simulink model "double_pendulum_model_2D"  (R2021a)
settings: Solver=FixedStepAuto  StartTime=0.0  StopTime=10.0  RelTol=1e-3
undefined symbols (not defined in the file): c1, c2, Cdp, g, l1, l2, mp1, mp2, mq, rho
settings Model: Creator=francois  LastModifiedBy=esl
settings SolverCC: AlgebraicLoopSolver=TrustRegion
settings DebuggingCC: SFMachineParentedDataDiag=warning

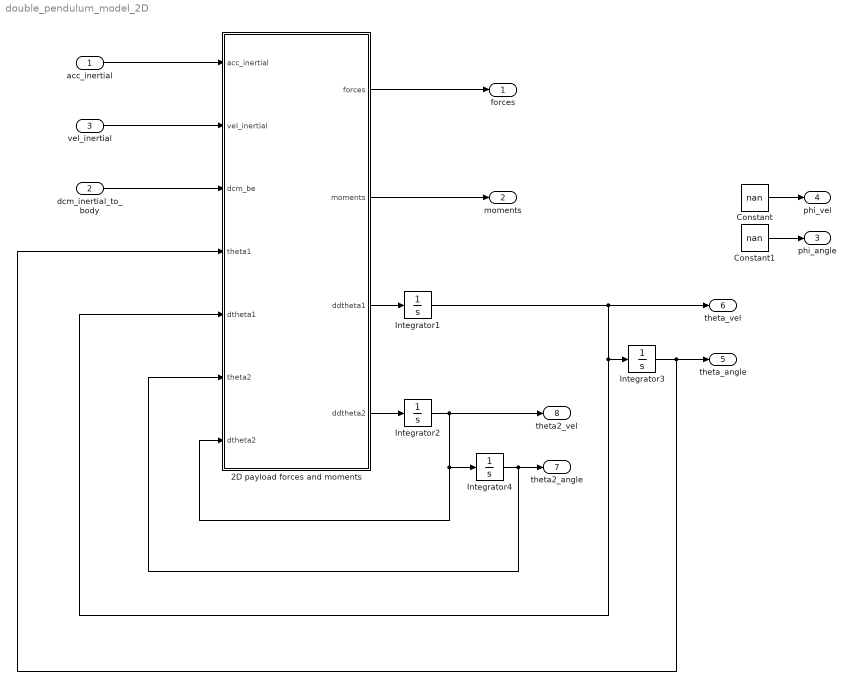
== system double_pendulum_model_2D ==
  acc_inertial : Inport  PortDimensions=3
  dcm_inertial_to_body : Inport  Port=2  PortDimensions=[3, 3]
  vel_inertial : Inport  Port=3  PortDimensions=3
  2D payload forces and moments : MATLAB Function  TreatAsAtomicUnit=on
  Constant : Constant  Value=nan
  Constant1 : Constant  Value=nan
  Integrator1 : Integrator
  Integrator2 : Integrator
  Integrator3 : Integrator  WrapState=on
  Integrator4 : Integrator  WrapState=on
  forces : Outport  PortDimensions=3
  moments : Outport  Port=2  PortDimensions=3
  phi_angle : Outport  Port=3  PortDimensions=1
  phi_vel : Outport  Port=4  PortDimensions=1
  theta_angle : Outport  Port=5  PortDimensions=1
  theta_vel : Outport  Port=6  PortDimensions=1
  theta2_angle : Outport  Port=7  PortDimensions=1
  theta2_vel : Outport  Port=8  PortDimensions=1
  wires:
  acc_inertial/1 -> 2D payload forces and moments/1(acc_inertial)
  dcm_inertial_to_body/1 -> 2D payload forces and moments/3(dcm_be)
  2D payload forces and moments/1(forces) -> forces/1
  Integrator1/1 -> 2D payload forces and moments/5(dtheta1), Integrator3/1, theta_vel/1
  2D payload forces and moments/3(ddtheta1) -> Integrator1/1
  Integrator3/1 -> 2D payload forces and moments/4(theta1), theta_angle/1
  2D payload forces and moments/2(moments) -> moments/1
  vel_inertial/1 -> 2D payload forces and moments/2(vel_inertial)
  Constant/1 -> phi_vel/1
  Constant1/1 -> phi_angle/1
  2D payload forces and moments/4(ddtheta2) -> Integrator2/1
  Integrator2/1 -> theta2_vel/1, 2D payload forces and moments/7(dtheta2), Integrator4/1
  Integrator4/1 -> 2D payload forces and moments/6(theta2), theta2_angle/1

== matlab function double_pendulum_model_2D/2D payload forces and moments ==
  data: acc_inertial input; vel_inertial input; forces output; dcm_be input; theta1 input; dtheta1 input; theta2 input; dtheta2 input; moments output; ddtheta1 output; ddtheta2 output; mq parameter; mp1 parameter; mp2 parameter; l1 parameter; l2 parameter; g parameter; c1 parameter; c2 parameter; Cdp parameter; rho parameter
function [forces, moments, ddtheta1 , ddtheta2] = double_pendulum_2D(acc_inertial, vel_inertial, dcm_be, theta1, dtheta1, theta2, dtheta2, mq, mp1, mp2, l1, l2, g, c1, c2, Cdp, rho)
    % all forces and states are relative to inertial frame coordinate frame
    
    % For variables used from MATLAB workspace, add them as function inputs
    % go to tab: "Editor", in section "SIMULINK", click "Edit Data"
    % for appropriate input args that are in MATLAB workspace, change scope
    % from "Input" to "Parameter"
    
    %% Drag forces
    fwt1 = (0.5*rho*(0 - ( vel_inertial(1) + dtheta1*l1*cos(theta1)                          ))^2*Cdp)*sign(vel_inertial(1));
    fwt2 = (0.5*rho*(0 - ( vel_inertial(1) + dtheta1*l1*cos(theta1) + dtheta2*l2*cos(theta2) ))^2*Cdp)*sign(vel_inertial(1));
    
    %% Quad acceleration    due to    actual payload angle and angular rate   
    % copy output from "calculate_double_pendulum_forces.m":
    ax = (2*fwt1*l1*l2*mp1^2 + 4*c1*dtheta1*l2*mp1^2*cos(theta1) + 2*fwt1*l1*l2*mp1*mp2 + 2*fwt1*l1*l2*mp1*mq + fwt1*l1*l2*mp2*mq + fwt2*l1*l2*mp1*mq + fwt2*l1*l2*mp2*mq + 2*fwt1*l1*l2*mp1^2*cos(2*theta1) + 2*g*l1*l2*mp1^2*mq*sin(2*theta1) + 4*c1*dtheta1*l2*mp1*mp2*cos(theta1) + 4*c1*dtheta1*l2*mp1*mq*cos(theta1) + 2*c1*dtheta1*l2*mp2*mq*cos(theta1) - 2*c2*dtheta1*l1*mp1*mq*cos(theta2) - 2*c2*dtheta1*l1*mp2*mq*cos(theta2) + 2*c2*dtheta2*l1*mp1*mq*cos(theta2) + 2*c2*dtheta2*l1*mp2*mq*cos(theta2) - 2*c1*dtheta1*l2*mp2*mq*cos(theta1 - 2*theta2) + 4*dtheta1^2*l1^2*l2*mp1^2*mq*sin(theta1) + 2*fwt1*l1*l2*mp1*mp2*cos(2*theta1) + 2*fwt1*l1*l2*mp1*mq*cos(2*theta1) + fwt1*l1*l2*mp2*mq*cos(2*theta1) - fwt2*l1*l2*mp1*mq*cos(2*theta1) - fwt1*l1*l2*mp2*mq*cos(2*theta2) + fwt2*l1*l2*mp1*mq*cos(2*theta2) - fwt2*l1*l2*mp2*mq*cos(2*theta1) + fwt2*l1*l2*mp2*mq*cos(2*theta2) + 2*c2*dtheta1*l1*mp1*mq*cos(2*theta1 - theta2) + 2*c2*dtheta1*l1*mp2*mq*cos(2*theta1 - theta2) - 2*c2*dtheta2*l1*mp1*mq*cos(2*theta1 - theta2) - 2*c2*dtheta2*l1*mp2*mq*cos(2*theta1 - theta2) - fwt1*l1*l2*mp2*mq*cos(2*theta1 - 2*theta2) - fwt2*l1*l2*mp1*mq*cos(2*theta1 - 2*theta2) - fwt2*l1*l2*mp2*mq*cos(2*theta1 - 2*theta2) + 2*dtheta2^2*l1*l2^2*mp1*mp2*mq*sin(2*theta1 - theta2) + 2*g*l1*l2*mp1*mp2*mq*sin(2*theta1) + 4*dtheta1^2*l1^2*l2*mp1*mp2*mq*sin(theta1) + 2*dtheta2^2*l1*l2^2*mp1*mp2*mq*sin(theta2))/(2*l1*l2*mq*(2*mp1*mp2 + 2*mp1*mq + mp2*mq + 2*mp1^2 - mp2*mq*cos(2*theta1 - 2*theta2)));
    az = (2*g*l1*l2*mp1^2*mq - 2*fwt1*l1*l2*mp1^2*sin(2*theta1) - 4*c1*dtheta1*l2*mp1^2*sin(theta1) + 2*g*l1*l2*mp1^2*mq*cos(2*theta1) - 4*c1*dtheta1*l2*mp1*mp2*sin(theta1) - 4*c1*dtheta1*l2*mp1*mq*sin(theta1) - 2*c1*dtheta1*l2*mp2*mq*sin(theta1) + 2*c2*dtheta1*l1*mp1*mq*sin(theta2) + 2*c2*dtheta1*l1*mp2*mq*sin(theta2) - 2*c2*dtheta2*l1*mp1*mq*sin(theta2) - 2*c2*dtheta2*l1*mp2*mq*sin(theta2) + 4*dtheta1^2*l1^2*l2*mp1^2*mq*cos(theta1) - 2*c1*dtheta1*l2*mp2*mq*sin(theta1 - 2*theta2) - 2*fwt1*l1*l2*mp1*mp2*sin(2*theta1) - 2*fwt1*l1*l2*mp1*mq*sin(2*theta1) - fwt1*l1*l2*mp2*mq*sin(2*theta1) + fwt2*l1*l2*mp1*mq*sin(2*theta1) + fwt1*l1*l2*mp2*mq*sin(2*theta2) - fwt2*l1*l2*mp1*mq*sin(2*theta2) + fwt2*l1*l2*mp2*mq*sin(2*theta1) - fwt2*l1*l2*mp2*mq*sin(2*theta2) + 2*g*l1*l2*mp1*mp2*mq - 2*c2*dtheta1*l1*mp1*mq*sin(2*theta1 - theta2) - 2*c2*dtheta1*l1*mp2*mq*sin(2*theta1 - theta2) + 2*c2*dtheta2*l1*mp1*mq*sin(2*theta1 - theta2) + 2*c2*dtheta2*l1*mp2*mq*sin(2*theta1 - theta2) - fwt1*l1*l2*mp2*mq*sin(2*theta1 - 2*theta2) + fwt2*l1*l2*mp1*mq*sin(2*theta1 - 2*theta2) + fwt2*l1*l2*mp2*mq*sin(2*theta1 - 2*theta2) + 2*dtheta2^2*l1*l2^2*mp1*mp2*mq*cos(2*theta1 - theta2) + 2*g*l1*l2*mp1*mp2*mq*cos(2*theta1) + 4*dtheta1^2*l1^2*l2*mp1*mp2*mq*cos(theta1) + 2*dtheta2^2*l1*l2^2*mp1*mp2*mq*cos(theta2))/(2*l1*l2*mq*(2*mp1*mp2 + 2*mp1*mq + mp2*mq + 2*mp1^2 - mp2*mq*cos(2*theta1 - 2*theta2)));

    ay = 0; % No y effect because using a 2D model
    
    %% Forces and moments based on payload contribution to acceleration
    forces = (mq + mp1 + mp2) * dcm_be * [ax; ay; az];
    moments = [0; 0; 0]; % No effect on moments
    
    %% Extract actual quad acceleration
    ddxq = acc_inertial(1);
%     ddy = acc_inertial(2); % No y effect because using a 2D model
    ddzq = acc_inertial(3);
        
    %% Payload angular acceleration,     due to    actual quad acceleration 
    % copy output from "calculate_double_pendulum_forces.m":
    ddtheta1 = -(c1*dtheta1*l2 + fwt1*l1*l2*cos(theta1) + c2*dtheta1*l1*cos(theta1 - theta2) - c2*dtheta2*l1*cos(theta1 - theta2) + (dtheta1^2*l1^2*l2*mp2*sin(2*theta1 - 2*theta2))/2 - fwt2*l1*l2*cos(theta1 - theta2)*cos(theta2) + ddxq*l1*l2*mp1*cos(theta1) + ddxq*l1*l2*mp2*cos(theta1) + dtheta2^2*l1*l2^2*mp2*sin(theta1 - theta2) - ddzq*l1*l2*mp1*sin(theta1) - ddzq*l1*l2*mp2*sin(theta1) + g*l1*l2*mp1*sin(theta1) + g*l1*l2*mp2*sin(theta1) - ddxq*l1*l2*mp2*cos(theta1 - theta2)*cos(theta2) + ddzq*l1*l2*mp2*cos(theta1 - theta2)*sin(theta2) - g*l1*l2*mp2*cos(theta1 - theta2)*sin(theta2))/(l1^2*l2*(mp1 + mp2 - mp2*cos(theta1 - theta2)^2));
    ddtheta2 = (2*c2*dtheta1*l1*mp1 + 2*c2*dtheta1*l1*mp2 - 2*c2*dtheta2*l1*mp1 - 2*c2*dtheta2*l1*mp2 + 2*c1*dtheta1*l2*mp2*cos(theta1 - theta2) - ddxq*l1*l2*mp2^2*cos(theta2) + 2*dtheta1^2*l1^2*l2*mp2^2*sin(theta1 - theta2) + ddzq*l1*l2*mp2^2*sin(theta2) - g*l1*l2*mp2^2*sin(theta2) + fwt1*l1*l2*mp2*cos(2*theta1 - theta2) + dtheta2^2*l1*l2^2*mp2^2*sin(2*theta1 - 2*theta2) + ddxq*l1*l2*mp2^2*cos(2*theta1 - theta2) + fwt1*l1*l2*mp2*cos(theta2) - 2*fwt2*l1*l2*mp1*cos(theta2) - 2*fwt2*l1*l2*mp2*cos(theta2) - ddzq*l1*l2*mp2^2*sin(2*theta1 - theta2) + g*l1*l2*mp2^2*sin(2*theta1 - theta2) - ddxq*l1*l2*mp1*mp2*cos(theta2) + 2*dtheta1^2*l1^2*l2*mp1*mp2*sin(theta1 - theta2) + ddzq*l1*l2*mp1*mp2*sin(theta2) - g*l1*l2*mp1*mp2*sin(theta2) + ddxq*l1*l2*mp1*mp2*cos(2*theta1 - theta2) - ddzq*l1*l2*mp1*mp2*sin(2*theta1 - theta2) + g*l1*l2*mp1*mp2*sin(2*theta1 - theta2))/(l1*l2^2*mp2*(2*mp1 + mp2 - mp2*cos(2*theta1 - 2*theta2)));

end
